simulink model "simulation"  (R2018a)
settings: Solver=VariableStepAuto  StartTime=0.0  StopTime=5  RelTol=1e-3
undefined symbols (not defined in the file): A, B, C, K, L
libraries: simulink x2
settings Model: Creator=Migue  LastModifiedBy=Migue

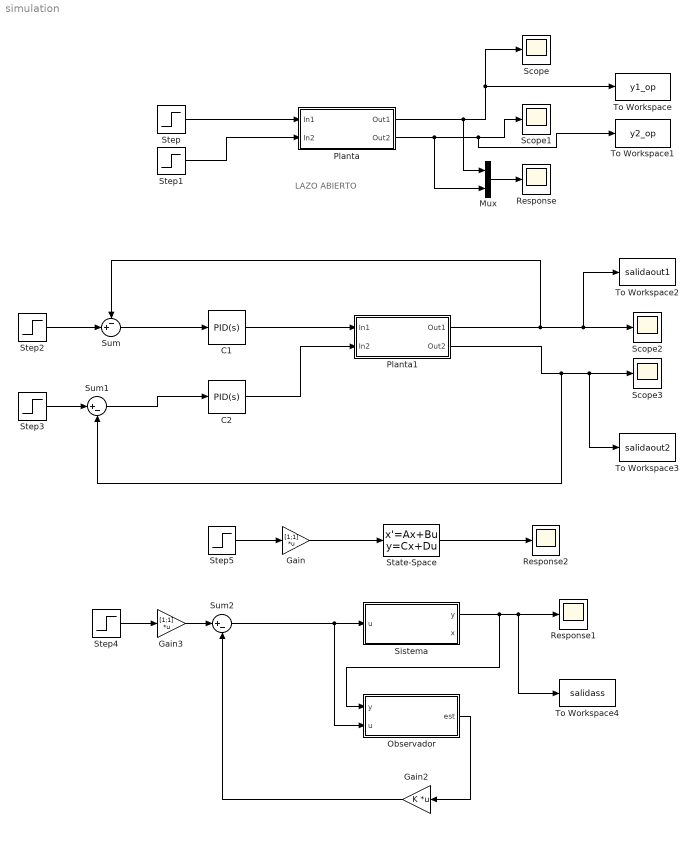
== system simulation ==
  note: LAZO ABIERTO
  C1 : simulink/Continuous/PID Controller  Controller=PID  TimeDomain=Continuous-time  SampleTime=-1  IntegratorMethod=Forward Euler  FilterMethod=Forward Euler  Form=Parallel  UseFilter=on  ControllerParametersSource=internal  P=81.85  I=1000.50  D=0  N=100  InitialConditionSource=internal  InitialConditionForIntegrator=0  InitialConditionForFilter=0  ExternalReset=none  LimitOutput=off  UpperSaturationLimit=inf  LowerSaturationLimit=-inf  LinearizeAsGain=on  AntiWindupMode=none  Kb=1  TrackingMode=off  Kt=1  PParamMin=[]  PParamMax=[]  IParamMin=[]  IParamMax=[]  DParamMin=[]  DParamMax=[]  NParamMin=[]  NParamMax=[]  KbParamMin=[]  KbParamMax=[]  KtParamMin=[]  KtParamMax=[]  POutMin=[]  POutMax=[]  IOutMin=[]  IOutMax=[]  DOutMin=[]  DOutMax=[]  NOutMin=[]  NOutMax=[]  KbOutMin=[]  KbOutMax=[]  KtOutMin=[]  KtOutMax=[]  IntegratorOutMin=[]  IntegratorOutMax=[]  FilterOutMin=[]  FilterOutMax=[]  SumOutMin=[]  SumOutMax=[]  SumI1OutMin=[]  SumI1OutMax=[]  SumI2OutMin=[]  SumI2OutMax=[]  SumI3OutMin=[]  SumI3OutMax=[]  SumDOutMin=[]  SumDOutMax=[]  SaturationOutMin=[]  SaturationOutMax=[]  IntegratorContinuousStateAttributes=''  IntegratorStateMustResolveToSignalObject=off  IntegratorRTWStateStorageClass=Auto  FilterContinuousStateAttributes=''  FilterStateMustResolveToSignalObject=off  FilterRTWStateStorageClass=Auto  DifferentiatorICPrevScaledInput=0  DifferentiatorOutMin=[]  DifferentiatorOutMax=[]  FilterDiffOutCoefMin=[]  FilterDiffOutCoefMax=[]  SumDenOutMin=[]  SumDenOutMax=[]  SumNumOutMin=[]  SumNumOutMax=[]  ReciprocalOutMin=[]  ReciprocalOutMax=[]  DivideOutMin=[]  DivideOutMax=[]  TunerSelectOption=Transfer Function Based (PID Tuner App)
  "C2 " : simulink/Continuous/PID Controller  Controller=PID  TimeDomain=Continuous-time  SampleTime=-1  IntegratorMethod=Forward Euler  FilterMethod=Forward Euler  Form=Parallel  UseFilter=on  ControllerParametersSource=internal  P=5  I=400  D=0  N=100  InitialConditionSource=internal  InitialConditionForIntegrator=0  InitialConditionForFilter=0  ExternalReset=none  LimitOutput=off  UpperSaturationLimit=inf  LowerSaturationLimit=-inf  LinearizeAsGain=on  AntiWindupMode=none  Kb=1  TrackingMode=off  Kt=1  PParamMin=[]  PParamMax=[]  IParamMin=[]  IParamMax=[]  DParamMin=[]  DParamMax=[]  NParamMin=[]  NParamMax=[]  KbParamMin=[]  KbParamMax=[]  KtParamMin=[]  KtParamMax=[]  POutMin=[]  POutMax=[]  IOutMin=[]  IOutMax=[]  DOutMin=[]  DOutMax=[]  NOutMin=[]  NOutMax=[]  KbOutMin=[]  KbOutMax=[]  KtOutMin=[]  KtOutMax=[]  IntegratorOutMin=[]  IntegratorOutMax=[]  FilterOutMin=[]  FilterOutMax=[]  SumOutMin=[]  SumOutMax=[]  SumI1OutMin=[]  SumI1OutMax=[]  SumI2OutMin=[]  SumI2OutMax=[]  SumI3OutMin=[]  SumI3OutMax=[]  SumDOutMin=[]  SumDOutMax=[]  SaturationOutMin=[]  SaturationOutMax=[]  IntegratorContinuousStateAttributes=''  IntegratorStateMustResolveToSignalObject=off  IntegratorRTWStateStorageClass=Auto  FilterContinuousStateAttributes=''  FilterStateMustResolveToSignalObject=off  FilterRTWStateStorageClass=Auto  DifferentiatorICPrevScaledInput=0  DifferentiatorOutMin=[]  DifferentiatorOutMax=[]  FilterDiffOutCoefMin=[]  FilterDiffOutCoefMax=[]  SumDenOutMin=[]  SumDenOutMax=[]  SumNumOutMin=[]  SumNumOutMax=[]  ReciprocalOutMin=[]  ReciprocalOutMax=[]  DivideOutMin=[]  DivideOutMax=[]  TunerSelectOption=Transfer Function Based (PID Tuner App)
  Gain : Gain  Gain=[1;1]  Multiplication=Matrix(K*u)
  Gain2 : Gain  Gain=K  Multiplication=Matrix(K*u)
  Gain3 : Gain  Gain=[1;1]  Multiplication=Matrix(K*u)
  Mux : Mux  Inputs=2
  Observador : Subsystem
  Planta : Subsystem
  Planta1 : Subsystem
  Response : Scope
  Response1 : Scope
  Response2 : Scope
  Scope{,1..3} (4 alike) : Scope
  Sistema : Subsystem
  State-Space : StateSpace  A=A  B=B  C=C  D=[0 0;0 0]  InitialCondition=0
  Step{,1..5} (6 alike) : Step  SampleTime=0
  Sum : Sum  Inputs=-+|
  Sum1 : Sum  Inputs=|+-
  Sum2 : Sum  Inputs=|+-
  To Workspace : ToWorkspace  VariableName=y1_op  SaveFormat=Timeseries  SampleTime=-1
  To Workspace1 : ToWorkspace  VariableName=y2_op  SaveFormat=Timeseries  SampleTime=-1
  To Workspace2 : ToWorkspace  VariableName=salidaout1  SaveFormat=Timeseries  SampleTime=-1
  To Workspace3 : ToWorkspace  VariableName=salidaout2  SaveFormat=Timeseries  SampleTime=-1
  To Workspace4 : ToWorkspace  VariableName=salidass  SaveFormat=Timeseries  SampleTime=-1
  wires:
  Step1/1 -> Planta/2(In2)
  Step/1 -> Planta/1(In1)
  Planta/2(Out2) -> Mux/2, To Workspace1/1, Scope1/1
  Planta/1(Out1) -> Mux/1, To Workspace/1, Scope/1
  Step3/1 -> Sum1/1
  Step2/1 -> Sum/2
  Planta1/2(Out2) -> Sum1/2, To Workspace3/1, Scope3/1
  Planta1/1(Out1) -> Sum/1, To Workspace2/1, Scope2/1
  C1/1 -> Planta1/1(In1)
  Sum/1 -> C1/1
  Sum1/1 -> "C2 "/1
  "C2 "/1 -> Planta1/2(In2)
  Mux/1 -> Response/1
  State-Space/1 -> Response2/1
  Step5/1 -> Gain/1
  Gain/1 -> State-Space/1
  Sum2/1 -> Observador/2(u), Sistema/1(u)
  Sistema/1(y) -> Observador/1(y), To Workspace4/1, Response1/1
  Observador/1(est) -> Gain2/1
  Step4/1 -> Gain3/1
  Gain3/1 -> Sum2/1
  Gain2/1 -> Sum2/2

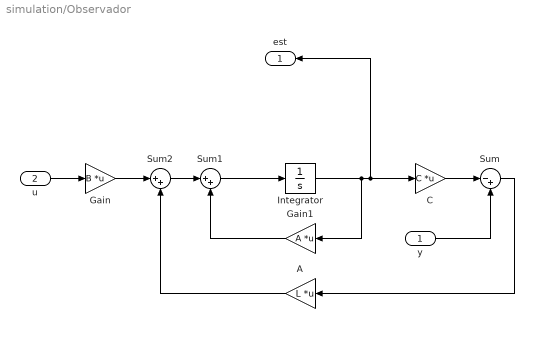
== system simulation/Observador ==
  y : Inport
  u : Inport  Port=2
  "A " : Gain  Gain=L  Multiplication=Matrix(K*u)
  C : Gain  Gain=C  Multiplication=Matrix(K*u)
  Gain : Gain  Gain=B  Multiplication=Matrix(K*u)
  Gain1 : Gain  Gain=A  Multiplication=Matrix(K*u)
  Integrator : Integrator
  Sum : Sum  Inputs=|-+
  Sum1 : Sum  Inputs=|++
  Sum2 : Sum  Inputs=|++
  est : Outport
  wires:
  u/1 -> Gain/1
  Sum1/1 -> Integrator/1
  Integrator/1 -> Gain1/1, est/1, C/1
  Gain1/1 -> Sum1/2
  Gain/1 -> Sum2/1
  Sum2/1 -> Sum1/1
  "A "/1 -> Sum2/2
  C/1 -> Sum/1
  y/1 -> Sum/2
  Sum/1 -> "A "/1

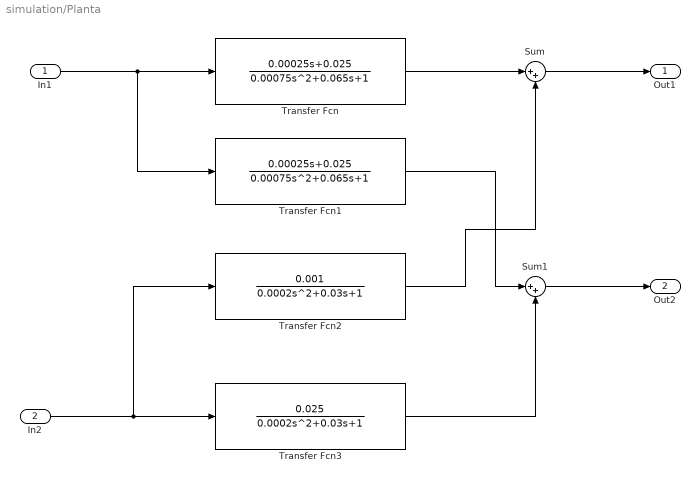
== system simulation/Planta ==
  In1 : Inport
  In2 : Inport  Port=2
  Sum : Sum  Inputs=|++
  Sum1 : Sum  Inputs=|++
  Transfer Fcn : TransferFcn  Numerator=[0.00025 0.025]  Denominator=[0.00075 0.065 1]
  Transfer Fcn1 : TransferFcn  Numerator=[0.00025 0.025]  Denominator=[0.00075 0.065 1]
  Transfer Fcn2 : TransferFcn  Numerator=[0.001]  Denominator=[0.0002 0.03 1]
  Transfer Fcn3 : TransferFcn  Numerator=[0.025]  Denominator=[0.0002 0.03 1]
  Out1 : Outport
  Out2 : Outport  Port=2
  wires:
  In1/1 -> Transfer Fcn1/1, Transfer Fcn/1
  In2/1 -> Transfer Fcn3/1, Transfer Fcn2/1
  Transfer Fcn1/1 -> Sum1/1
  Transfer Fcn/1 -> Sum/1
  Transfer Fcn2/1 -> Sum/2
  Sum/1 -> Out1/1
  Transfer Fcn3/1 -> Sum1/2
  Sum1/1 -> Out2/1

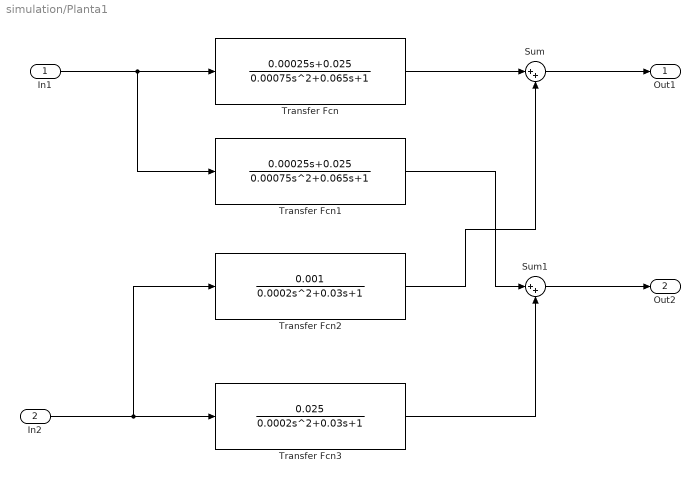
== system simulation/Planta1 ==
  In1 : Inport
  In2 : Inport  Port=2
  Sum : Sum  Inputs=|++
  Sum1 : Sum  Inputs=|++
  Transfer Fcn : TransferFcn  Numerator=[0.00025 0.025]  Denominator=[0.00075 0.065 1]
  Transfer Fcn1 : TransferFcn  Numerator=[0.00025 0.025]  Denominator=[0.00075 0.065 1]
  Transfer Fcn2 : TransferFcn  Numerator=[0.001]  Denominator=[0.0002 0.03 1]
  Transfer Fcn3 : TransferFcn  Numerator=[0.025]  Denominator=[0.0002 0.03 1]
  Out1 : Outport
  Out2 : Outport  Port=2
  wires:
  In1/1 -> Transfer Fcn1/1, Transfer Fcn/1
  In2/1 -> Transfer Fcn3/1, Transfer Fcn2/1
  Transfer Fcn1/1 -> Sum1/1
  Transfer Fcn/1 -> Sum/1
  Transfer Fcn2/1 -> Sum/2
  Sum/1 -> Out1/1
  Transfer Fcn3/1 -> Sum1/2
  Sum1/1 -> Out2/1

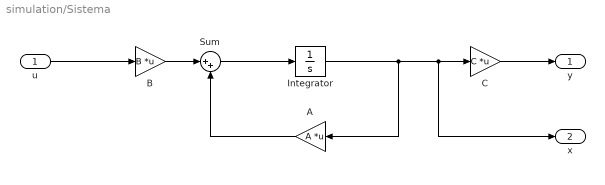
== system simulation/Sistema ==
  u : Inport
  A : Gain  Gain=A  Multiplication=Matrix(K*u)
  B : Gain  Gain=B  Multiplication=Matrix(K*u)
  C : Gain  Gain=C  Multiplication=Matrix(K*u)
  Integrator : Integrator
  Sum : Sum  Inputs=|++
  y : Outport
  x : Outport  Port=2
  wires:
  u/1 -> B/1
  B/1 -> Sum/1
  Sum/1 -> Integrator/1
  C/1 -> y/1
  Integrator/1 -> A/1, x/1, C/1
  A/1 -> Sum/2
